simulink model "PrviZadatakSimulacija"  (R2018a)
settings: Solver=VariableStepAuto  StartTime=0.0  StopTime=10.0  RelTol=1e-3
values from neighbouring files (symbols this model uses):
  k = sqrt(1+x2^2)    [prviZadatak-potencijalno resenje.m]    (also in prviZadatak2RADI.m)
  x2 = 100    [prviZadatak-potencijalno resenje.m]    (also in prviZadatak2RADI.m = cos(3*pi*t2))
settings Model: Creator=Asus  LastModifiedBy=Asus

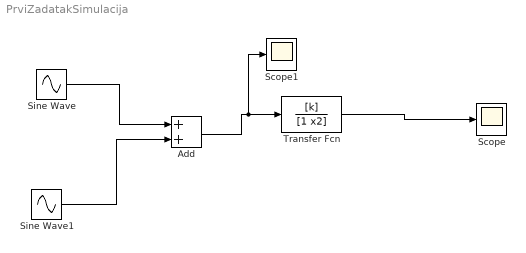
== system PrviZadatakSimulacija ==
  Add : Sum
  Scope : Scope
  Scope1 : Scope
  Sine Wave : Sin  Frequency=3*pi  Phase=pi/2  SampleTime=0
  Sine Wave1 : Sin  Frequency=1500*pi  SampleTime=0
  Transfer Fcn : TransferFcn  Numerator=[k]  Denominator=[1 x2]
  wires:
  Sine Wave/1 -> Add/1
  Sine Wave1/1 -> Add/2
  Add/1 -> Scope1/1, Transfer Fcn/1
  Transfer Fcn/1 -> Scope/1
